simulink model "gm_CustArch_v2_vnl"  (R2020a)
settings: Solver=FixedStepDiscrete  StartTime=0.0  StopTime=840000  RelTol=1e-3
libraries: simulink x172, hdlsllib x102
(part 1 of 4)
settings Model: FPTRunName=FPA_Reference  PacingRate=71  Creator=BuccelliLab  LastModifiedBy=diflo
settings SolverCC: AutoInsertRateTranBlk=on  MinimalZcImpactIntegration=on
settings DataIOCC: LimitDataPoints=on  SaveOutput=off  SaveTime=off  ReturnWorkspaceOutputs=off
settings OptimizationCC: BlockReduction=off  ConditionallyExecuteInputs=off  DefaultParameterBehavior=Inlined  LifeSpan=inf
settings DebuggingCC: SignalRangeChecking=warning  ReadBeforeWriteMsg=DisableAll  WriteAfterWriteMsg=DisableAll  WriteAfterReadMsg=DisableAll  AlgebraicLoopMsg=error  InheritedTsInSrcMsg=none  MultiTaskDSMMsg=none  SingleTaskRateTransMsg=error  ParameterDowncastMsg=warning  ParameterOverflowMsg=warning  AllowSymbolicDim=off  StrictBusMsg=ErrorOnBusTreatedAsVector  SFUnexpectedBacktrackingDiag=warning  SFNoUnconditionalDefaultTransitionDiag=warning  SFExecutionAtInitializationDiag=none  ArithmeticOperatorsInVariantConditions=warning
settings HardwareCC: ProdBitPerPointer=32  ProdBitPerSizeT=32  ProdBitPerPtrDiffT=32  ProdLargestAtomicFloat=None  ProdIntDivRoundTo=Undefined  ProdEndianess=Unspecified  ProdWordSize=32  ProdHWDeviceType=ASIC/FPGA->ASIC/FPGA  TargetBitPerPointer=64  TargetBitPerSizeT=64  TargetBitPerPtrDiffT=64  TargetLongLongMode=on  TargetIntDivRoundTo=Zero  TargetEndianess=LittleEndian  TargetWordSize=64  TargetHWDeviceType=Custom Processor->MATLAB Host Computer  ProdEqTarget=off
settings ModelReferenceCC: UpdateModelReferenceTargets=IfOutOfDate
settings SFSimCC: SFSimEcho=off  SimUseLocalCustomCode=off  CustomCodeUndefinedFunction=UseInterfaceOnly
settings RTWCC: RTWUseLocalCustomCode=off
settings CodeAppCC: StateflowObjectComments=on
settings GRTTargetCC: TargetLangStandard=C89/C90 (ANSI)
settings ConfigComp: CovScope=ReferencedModels  CovMetricSettings=dw  CovHtmlReporting=on  CovSaveCumulativeToWorkspaceVar=on  CovSaveSingleToWorkspaceVar=on  CovExternalEMLEnable=off  CovSFcnEnable=off

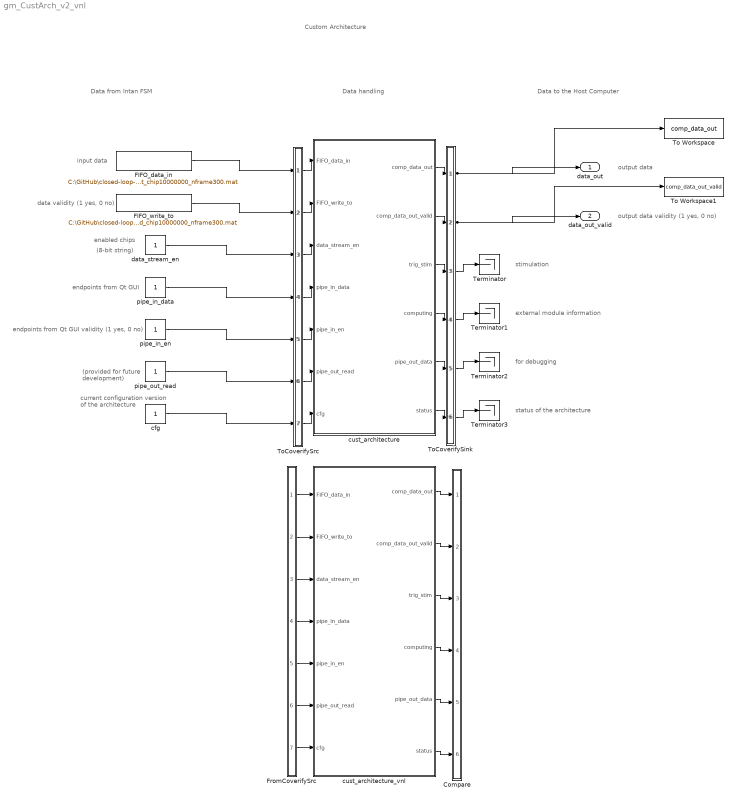
== system gm_CustArch_v2_vnl ==
  note: Data handling
  note: Custom Architecture
  note: output data validity (1 yes, 0 no)
  note: endpoints from Qt GUI
  note: (8-bit string)
  note: enabled chips
  note: data validity (1 yes, 0 no)
  note: input data
  note: endpoints from Qt GUI validity (1 yes, 0 no)
  note: (provided for future
      | development)
  note: current configuration
      | version of the
      | architecture
  note: output data
  note: Data to the Host Computer
  note: stimulation
  note: external module information
  note: for debugging
  note: status of the architecture
  note: Data from Intan FSM
  Compare : Subsystem
      mask Display: disp('')
  FIFO_data_in : FromFile  FileName=C:\GitHub\closed-loop-neuroscience\Mattia\Custom_architecture\CustArch_debug\fsm_out_chip10000000_nframe300.mat  OutDataTypeStr=uint16  SampleTime=1  ExtrapolationBeforeFirstDataPoint=Hold first value  InterpolationWithinTimeRange=Zero order hold  ExtrapolationAfterLastDataPoint=Hold last value
  FIFO_write_to : FromFile  FileName=C:\GitHub\closed-loop-neuroscience\Mattia\Custom_architecture\CustArch_debug\fsm_valid_chip10000000_nframe300.mat  OutDataTypeStr=boolean  SampleTime=1
  FromCoverifySrc : Subsystem
      mask Display: disp('')
  Terminator{,1..3} (4 alike) : Terminator
  To Workspace : ToWorkspace  VariableName=comp_data_out  SaveFormat=Timeseries  SampleTime=-1
  To Workspace1 : ToWorkspace  VariableName=comp_data_out_valid  SaveFormat=Timeseries  SampleTime=-1
  ToCoverifySink : Subsystem
      mask Display: disp('')
  ToCoverifySrc : Subsystem
      mask Display: disp('')
  cfg : Constant  OutDataTypeStr=uint16  SampleTime=-1
  cust_architecture : Subsystem
  cust_architecture_vnl : Subsystem
  data_stream_en : Constant  OutDataTypeStr=uint8  SampleTime=-1
  pipe_in_data : Constant  OutDataTypeStr=uint16  SampleTime=-1
  pipe_in_en : Constant  OutDataTypeStr=boolean  SampleTime=-1
  pipe_out_read : Constant  OutDataTypeStr=boolean  SampleTime=-1
  data_out : Outport  VectorParamsAs1DForOutWhenUnconnected=off
  data_out_valid : Outport  Port=2  VectorParamsAs1DForOutWhenUnconnected=off
  wires:
  ToCoverifySrc/1(out1) -> cust_architecture/1(FIFO_data_in)
  ToCoverifySrc/2(out2) -> cust_architecture/2(FIFO_write_to)
  ToCoverifySrc/3(out3) -> cust_architecture/3(data_stream_en)
  ToCoverifySrc/4(out4) -> cust_architecture/4(pipe_in_data)
  ToCoverifySrc/5(out5) -> cust_architecture/5(pipe_in_en)
  ToCoverifySrc/6(out6) -> cust_architecture/6(pipe_out_read)
  ToCoverifySrc/7(out7) -> cust_architecture/7(cfg)
  cust_architecture/1(comp_data_out) -> ToCoverifySink/1(in1)
  cust_architecture/2(comp_data_out_valid) -> ToCoverifySink/2(in2)
  cust_architecture/3(trig_stim) -> ToCoverifySink/3(in3)
  cust_architecture/4(computing) -> ToCoverifySink/4(in4)
  cust_architecture/5(pipe_out_data) -> ToCoverifySink/5(in5)
  cust_architecture/6(status) -> ToCoverifySink/6(in6)
  FIFO_data_in/1 -> ToCoverifySrc/1(in1)
  FIFO_write_to/1 -> ToCoverifySrc/2(in2)
  data_stream_en/1 -> ToCoverifySrc/3(in3)
  pipe_in_data/1 -> ToCoverifySrc/4(in4)
  pipe_in_en/1 -> ToCoverifySrc/5(in5)
  pipe_out_read/1 -> ToCoverifySrc/6(in6)
  cfg/1 -> ToCoverifySrc/7(in7)
  ToCoverifySink/1(out1) -> data_out/1, To Workspace/1
  ToCoverifySink/2(out2) -> data_out_valid/1, To Workspace1/1
  ToCoverifySink/3(out3) -> Terminator/1
  ToCoverifySink/4(out4) -> Terminator1/1
  ToCoverifySink/5(out5) -> Terminator2/1
  ToCoverifySink/6(out6) -> Terminator3/1
  FromCoverifySrc/1(out1) -> cust_architecture_vnl/1(FIFO_data_in)
  FromCoverifySrc/2(out2) -> cust_architecture_vnl/2(FIFO_write_to)
  FromCoverifySrc/3(out3) -> cust_architecture_vnl/3(data_stream_en)
  FromCoverifySrc/4(out4) -> cust_architecture_vnl/4(pipe_in_data)
  FromCoverifySrc/5(out5) -> cust_architecture_vnl/5(pipe_in_en)
  FromCoverifySrc/6(out6) -> cust_architecture_vnl/6(pipe_out_read)
  FromCoverifySrc/7(out7) -> cust_architecture_vnl/7(cfg)
  cust_architecture_vnl/1(comp_data_out) -> Compare/1(in1)
  cust_architecture_vnl/2(comp_data_out_valid) -> Compare/2(in2)
  cust_architecture_vnl/3(trig_stim) -> Compare/3(in3)
  cust_architecture_vnl/4(computing) -> Compare/4(in4)
  cust_architecture_vnl/5(pipe_out_data) -> Compare/5(in5)
  cust_architecture_vnl/6(status) -> Compare/6(in6)

== system gm_CustArch_v2_vnl/Compare ==
  in1 : Inport
  in2 : Inport  Port=2
  in3 : Inport  Port=3
  in4 : Inport  Port=4
  in5 : Inport  Port=5
  in6 : Inport  Port=6
  Assert_comp_data_out : Subsystem
  Assert_comp_data_out_valid : Subsystem
  Assert_computing : Subsystem
  Assert_pipe_out_data : Subsystem
  Assert_status : Subsystem
  Assert_trig_stim : Subsystem
  CleanupScopes : Subsystem
      settings: OpenFcn=|
      | blkName = gcb; %self block
      | idx = regexp(blkName, '/CleanupScopes$', 'once');
      | blkParent = blkName(1:idx-1);
      | blks=find_system(blkParent, 'LookUnderMasks', 'all','blocktype', 'Scope');
      | for itr = 1:length(blks)
      | 	 hScopeCfg = get_param(blks{itr},'ScopeConfiguration');
      | 	 hScopeCfg.Visible = ~ hScopeCfg.Visible;
      | end
      | drawnow;
      mask Display: fprintf(message('hdlcoder:cosim:vnl_dblclick').getString());
  Enable : Subsystem
      settings: OpenFcn=|
      | blkName = gcb;
      | idx = regexp(blkName, '/Enable$', 'once');
      | blkParent = blkName(1:idx-1);
      | blks=find_system(blkParent, 'LookUnderMasks', 'all','blocktype', 'Assertion');
      | e = get_param(blks{1}, 'Enabled');
      | if strcmp(e, 'on'), f= 'off';, else, f = 'on';, end
      | for ii=1:length(blks), set_param(blks{ii}, 'Enabled', f);, end
      | set_param(gcb, 'MaskDisplay',['fprintf(message(''hdlcoder:cosim:vnl_dblclick_assertions'',','''',upper(e),'''',').getString())']);
      mask Display: fprintf(message('hdlcoder:cosim:vnl_dblclick_assertions','OFF').getString());
  wires:
  in1/1 -> Assert_comp_data_out/1(cosim)
  [out1] -> Assert_comp_data_out/2(dut)
  in2/1 -> Assert_comp_data_out_valid/1(cosim)
  [out2] -> Assert_comp_data_out_valid/2(dut)
  in3/1 -> Assert_trig_stim/1(cosim)
  [out3] -> Assert_trig_stim/2(dut)
  in4/1 -> Assert_computing/1(cosim)
  [out4] -> Assert_computing/2(dut)
  in5/1 -> Assert_pipe_out_data/1(cosim)
  [out5] -> Assert_pipe_out_data/2(dut)
  in6/1 -> Assert_status/1(cosim)
  [out6] -> Assert_status/2(dut)

== system gm_CustArch_v2_vnl/FromCoverifySrc ==
  out1 : Outport
  out2 : Outport  Port=2
  out3 : Outport  Port=3
  out4 : Outport  Port=4
  out5 : Outport  Port=5
  out6 : Outport  Port=6
  out7 : Outport  Port=7
  wires:
  [in1] -> out1/1
  [in2] -> out2/1
  [in3] -> out3/1
  [in4] -> out4/1
  [in5] -> out5/1
  [in6] -> out6/1
  [in7] -> out7/1

== system gm_CustArch_v2_vnl/ToCoverifySink ==
  in1 : Inport
  in2 : Inport  Port=2
  in3 : Inport  Port=3
  in4 : Inport  Port=4
  in5 : Inport  Port=5
  in6 : Inport  Port=6
  out1 : Outport
  out2 : Outport  Port=2
  out3 : Outport  Port=3
  out4 : Outport  Port=4
  out5 : Outport  Port=5
  out6 : Outport  Port=6
  tag scope: out1=global, out2=global, out3=global, out4=global, out5=global, out6=global
  wires:
  in1/1 -> out1/1, [out1]
  in2/1 -> out2/1, [out2]
  in3/1 -> out3/1, [out3]
  in4/1 -> out4/1, [out4]
  in5/1 -> out5/1, [out5]
  in6/1 -> out6/1, [out6]

== system gm_CustArch_v2_vnl/ToCoverifySrc ==
  in1 : Inport
  in2 : Inport  Port=2
  in3 : Inport  Port=3
  in4 : Inport  Port=4
  in5 : Inport  Port=5
  in6 : Inport  Port=6
  in7 : Inport  Port=7
  out1 : Outport
  out2 : Outport  Port=2
  out3 : Outport  Port=3
  out4 : Outport  Port=4
  out5 : Outport  Port=5
  out6 : Outport  Port=6
  out7 : Outport  Port=7
  tag scope: in1=global, in2=global, in3=global, in4=global, in5=global, in6=global, in7=global
  wires:
  in1/1 -> out1/1, [in1]
  in2/1 -> out2/1, [in2]
  in3/1 -> out3/1, [in3]
  in4/1 -> out4/1, [in4]
  in5/1 -> out5/1, [in5]
  in6/1 -> out6/1, [in6]
  in7/1 -> out7/1, [in7]

== system gm_CustArch_v2_vnl/cust_architecture ==
  FIFO_data_in : Inport  OutDataTypeStr=uint16  PortDimensions=1  SampleTime=1
  FIFO_write_to : Inport  Port=2  OutDataTypeStr=boolean  PortDimensions=1  SampleTime=1
  data_stream_en : Inport  Port=3  OutDataTypeStr=uint8  PortDimensions=1  SampleTime=1
  pipe_in_data : Inport  Port=4  OutDataTypeStr=uint16  PortDimensions=1  SampleTime=1
  pipe_in_en : Inport  Port=5  OutDataTypeStr=boolean  PortDimensions=1  SampleTime=1
  pipe_out_read : Inport  Port=6  OutDataTypeStr=boolean  PortDimensions=1  SampleTime=1
  cfg : Inport  Port=7  OutDataTypeStr=uint16  PortDimensions=1  SampleTime=1
  Constant : Constant  OutDataTypeStr=uint8  SampleTime=1
  Constant1 : Constant  OutDataTypeStr=boolean  SampleTime=1
  Constant2 : Constant  OutDataTypeStr=uint16  SampleTime=1
  Constant3 : Constant  OutDataTypeStr=uint16  SampleTime=1
  Terminator2 : Terminator
  Terminator3 : Terminator
  Terminator4 : Terminator
  collect_output : Subsystem
  input_interpret_store_retrieve : Subsystem
  output_interpret : Subsystem
  pipe_in_interpret : Subsystem
  process_and_retrieve : Subsystem
  comp_data_out : Outport  VectorParamsAs1DForOutWhenUnconnected=off
  comp_data_out_valid : Outport  Port=2  OutDataTypeStr=boolean  VectorParamsAs1DForOutWhenUnconnected=off
  trig_stim : Outport  Port=3  VectorParamsAs1DForOutWhenUnconnected=off
  computing : Outport  Port=4  VectorParamsAs1DForOutWhenUnconnected=off
  pipe_out_data : Outport  Port=5  VectorParamsAs1DForOutWhenUnconnected=off
  status : Outport  Port=6  VectorParamsAs1DForOutWhenUnconnected=off
  wires:
  process_and_retrieve/1(rd_dout) -> collect_output/8(rd_dout)
  pipe_in_interpret/1(Out1) -> process_and_retrieve/5(value_from_pipeIn)
  output_interpret/3(read_address) -> input_interpret_store_retrieve/3(read_address), collect_output/6(rd_address)
  output_interpret/2(rd_enable) -> collect_output/5(rd_enable)
  output_interpret/1(OutputState) -> collect_output/4(OutputState)
  input_interpret_store_retrieve/4(read_from_processing_addr) -> process_and_retrieve/4(read_from_processing_addr)
  input_interpret_store_retrieve/3(current_value) -> process_and_retrieve/3(current_value)
  input_interpret_store_retrieve/2(read_from_storage_value) -> collect_output/7(read_from_storage_value)
  input_interpret_store_retrieve/1(InputState) -> process_and_retrieve/2(InputState), output_interpret/2(InputState), collect_output/3(InputState)
  collect_output/3(rd_address_bit_set_AC_during_DC) -> process_and_retrieve/1(rd_address_bit_set_AC_during_DC)
  collect_output/2(comp_data_out) -> comp_data_out/1
  collect_output/1(comp_data_out_valid) -> comp_data_out_valid/1
  Constant3/1 -> status/1
  Constant2/1 -> pipe_out_data/1
  Constant1/1 -> computing/1
  Constant/1 -> trig_stim/1
  cfg/1 -> Terminator2/1
  pipe_out_read/1 -> Terminator3/1
  pipe_in_en/1 -> Terminator4/1
  pipe_in_data/1 -> pipe_in_interpret/1(In1)
  data_stream_en/1 -> input_interpret_store_retrieve/4(data_stream_enable), output_interpret/1(data_stream_enable)
  FIFO_write_to/1 -> input_interpret_store_retrieve/2(FIFO_write_to), collect_output/2(FIFO_write_to)
  FIFO_data_in/1 -> collect_output/1(FIFO_data_in), input_interpret_store_retrieve/1(FIFO_data_in)

== system gm_CustArch_v2_vnl/cust_architecture_vnl ==
  note: Input
  note: Output
  note: Processing
  note: Unused
  FIFO_data_in : Inport
  FIFO_write_to : Inport  Port=2
  data_stream_en : Inport  Port=3
  pipe_in_data : Inport  Port=4
  pipe_in_en : Inport  Port=5
  pipe_out_read : Inport  Port=6
  cfg : Inport  Port=7
  Constant : Constant  OutDataTypeStr=uint8  SampleTime=-1
  Constant1 : Constant  OutDataTypeStr=boolean  SampleTime=-1
  Constant2 : Constant  OutDataTypeStr=uint16  SampleTime=-1
  Constant3 : Constant  OutDataTypeStr=uint16  SampleTime=-1
  Terminator2 : Terminator
  Terminator3 : Terminator
  Terminator4 : Terminator
  collect_output : Subsystem
  input_interpret_store_retrieve : Subsystem
  output_interpret : Subsystem
  pipe_in_interpret : Subsystem
  process_and_retrieve : Subsystem
  comp_data_out : Outport  VectorParamsAs1DForOutWhenUnconnected=off
  comp_data_out_valid : Outport  Port=2  OutDataTypeStr=boolean  VectorParamsAs1DForOutWhenUnconnected=off
  trig_stim : Outport  Port=3  VectorParamsAs1DForOutWhenUnconnected=off
  computing : Outport  Port=4  VectorParamsAs1DForOutWhenUnconnected=off
  pipe_out_data : Outport  Port=5  VectorParamsAs1DForOutWhenUnconnected=off
  status : Outport  Port=6  VectorParamsAs1DForOutWhenUnconnected=off
  wires:
  process_and_retrieve/1(rd_dout) -> collect_output/8(rd_dout)
  pipe_in_interpret/1(Out1) -> process_and_retrieve/5(value_from_pipeIn)
  input_interpret_store_retrieve/4(read_from_processing_addr) -> process_and_retrieve/4(read_from_processing_addr)
  input_interpret_store_retrieve/3(current_value) -> process_and_retrieve/3(current_value)
  collect_output/3(rd_address_bit_set_AC_during_DC) -> process_and_retrieve/1(rd_address_bit_set_AC_during_DC)
  pipe_in_data/1 -> pipe_in_interpret/1(In1)
  output_interpret/2(rd_enable) -> collect_output/5(rd_enable)
  output_interpret/1(OutputState) -> collect_output/4(OutputState)
  output_interpret/3(read_address) -> input_interpret_store_retrieve/3(read_address), collect_output/6(rd_address)
  input_interpret_store_retrieve/2(read_from_storage_value) -> collect_output/7(read_from_storage_value)
  input_interpret_store_retrieve/1(InputState) -> process_and_retrieve/2(InputState), output_interpret/2(InputState), collect_output/3(InputState)
  collect_output/2(comp_data_out) -> comp_data_out/1
  collect_output/1(comp_data_out_valid) -> comp_data_out_valid/1
  pipe_in_en/1 -> Terminator4/1
  pipe_out_read/1 -> Terminator3/1
  cfg/1 -> Terminator2/1
  Constant3/1 -> status/1
  Constant2/1 -> pipe_out_data/1
  Constant1/1 -> computing/1
  Constant/1 -> trig_stim/1
  data_stream_en/1 -> input_interpret_store_retrieve/4(data_stream_enable), output_interpret/1(data_stream_enable)
  FIFO_write_to/1 -> input_interpret_store_retrieve/2(FIFO_write_to), collect_output/2(FIFO_write_to)
  FIFO_data_in/1 -> collect_output/1(FIFO_data_in), input_interpret_store_retrieve/1(FIFO_data_in)

== system gm_CustArch_v2_vnl/Compare/Assert_comp_data_out ==
  cosim : Inport
  dut : Inport  Port=2
  AssertEq : Assertion  StopWhenAssertionFail=off
  Compare To Zero : simulink/Logic and Bit Operations/Compare To Zero  relop===  OutDataTypeStr=boolean
  Relational Operator : RelationalOperator  Operator===  OutDataTypeStr=boolean  RndMeth=Nearest
  compare: comp_data_out : Scope  NumInputPorts=3
  wires:
  Compare To Zero/1 -> compare: comp_data_out/3  "err"
  Relational Operator/1 -> Compare To Zero/1, AssertEq/1
  cosim/1 -> compare: comp_data_out/1, Relational Operator/1  "cosim"
  dut/1 -> compare: comp_data_out/2, Relational Operator/2  "dut ref"

== system gm_CustArch_v2_vnl/Compare/Assert_comp_data_out_valid ==
  cosim : Inport
  dut : Inport  Port=2
  AssertEq : Assertion  StopWhenAssertionFail=off
  Compare To Zero : simulink/Logic and Bit Operations/Compare To Zero  relop===  OutDataTypeStr=boolean
  Relational Operator : RelationalOperator  Operator===  OutDataTypeStr=boolean  RndMeth=Nearest
  compare: comp_data_out_valid : Scope  NumInputPorts=3
  wires:
  Compare To Zero/1 -> compare: comp_data_out_valid/3  "err"
  Relational Operator/1 -> Compare To Zero/1, AssertEq/1
  cosim/1 -> compare: comp_data_out_valid/1, Relational Operator/1  "cosim"
  dut/1 -> compare: comp_data_out_valid/2, Relational Operator/2  "dut ref"

== system gm_CustArch_v2_vnl/Compare/Assert_computing ==
  cosim : Inport
  dut : Inport  Port=2
  AssertEq : Assertion  StopWhenAssertionFail=off
  Compare To Zero : simulink/Logic and Bit Operations/Compare To Zero  relop===  OutDataTypeStr=boolean
  Relational Operator : RelationalOperator  Operator===  OutDataTypeStr=boolean  RndMeth=Nearest
  compare: computing : Scope  NumInputPorts=3
  wires:
  Compare To Zero/1 -> compare: computing/3  "err"
  Relational Operator/1 -> Compare To Zero/1, AssertEq/1
  cosim/1 -> compare: computing/1, Relational Operator/1  "cosim"
  dut/1 -> compare: computing/2, Relational Operator/2  "dut ref"

== system gm_CustArch_v2_vnl/Compare/Assert_pipe_out_data ==
  cosim : Inport
  dut : Inport  Port=2
  AssertEq : Assertion  StopWhenAssertionFail=off
  Compare To Zero : simulink/Logic and Bit Operations/Compare To Zero  relop===  OutDataTypeStr=boolean
  Relational Operator : RelationalOperator  Operator===  OutDataTypeStr=boolean  RndMeth=Nearest
  compare: pipe_out_data : Scope  NumInputPorts=3
  wires:
  Compare To Zero/1 -> compare: pipe_out_data/3  "err"
  Relational Operator/1 -> Compare To Zero/1, AssertEq/1
  cosim/1 -> compare: pipe_out_data/1, Relational Operator/1  "cosim"
  dut/1 -> compare: pipe_out_data/2, Relational Operator/2  "dut ref"

== system gm_CustArch_v2_vnl/Compare/Assert_status ==
  cosim : Inport
  dut : Inport  Port=2
  AssertEq : Assertion  StopWhenAssertionFail=off
  Compare To Zero : simulink/Logic and Bit Operations/Compare To Zero  relop===  OutDataTypeStr=boolean
  Relational Operator : RelationalOperator  Operator===  OutDataTypeStr=boolean  RndMeth=Nearest
  compare: status : Scope  NumInputPorts=3
  wires:
  Compare To Zero/1 -> compare: status/3  "err"
  Relational Operator/1 -> Compare To Zero/1, AssertEq/1
  cosim/1 -> compare: status/1, Relational Operator/1  "cosim"
  dut/1 -> compare: status/2, Relational Operator/2  "dut ref"

== system gm_CustArch_v2_vnl/Compare/Assert_trig_stim ==
  cosim : Inport
  dut : Inport  Port=2
  AssertEq : Assertion  StopWhenAssertionFail=off
  Compare To Zero : simulink/Logic and Bit Operations/Compare To Zero  relop===  OutDataTypeStr=boolean
  Relational Operator : RelationalOperator  Operator===  OutDataTypeStr=boolean  RndMeth=Nearest
  compare: trig_stim : Scope  NumInputPorts=3
  wires:
  Compare To Zero/1 -> compare: trig_stim/3  "err"
  Relational Operator/1 -> Compare To Zero/1, AssertEq/1
  cosim/1 -> compare: trig_stim/1, Relational Operator/1  "cosim"
  dut/1 -> compare: trig_stim/2, Relational Operator/2  "dut ref"

== system gm_CustArch_v2_vnl/Compare/CleanupScopes ==

== system gm_CustArch_v2_vnl/Compare/Enable ==

== system gm_CustArch_v2_vnl/cust_architecture/collect_output ==
  FIFO_data_in : Inport  OutDataTypeStr=uint16  PortDimensions=1  SampleTime=1
  FIFO_write_to : Inport  Port=2  OutDataTypeStr=boolean  PortDimensions=1  SampleTime=1
  InputState : Inport  Port=3  OutDataTypeStr=uint8  PortDimensions=1  SampleTime=1
  OutputState : Inport  Port=4  OutDataTypeStr=uint8  PortDimensions=1  SampleTime=1
  rd_enable : Inport  Port=5  OutDataTypeStr=boolean  PortDimensions=1  SampleTime=1
  rd_address : Inport  Port=6  OutDataTypeStr=fixdt(0, 9, 0)  PortDimensions=1  SampleTime=1
  read_from_storage_value : Inport  Port=7  OutDataTypeStr=uint16  PortDimensions=1  SampleTime=1
  rd_dout : Inport  Port=8  OutDataTypeStr=uint16  PortDimensions=1  SampleTime=1
  AND : Logic  AllPortsSameDT=off  OutDataTypeStr=boolean  SampleTime=1
  Bit Set to get AC during DC : simulink/Logic and Bit Operations/Bit Set  iBit=0
      settings: SourceProductBaseCode=SL
  Compare To Constant : simulink/Logic and Bit Operations/Compare To Constant  relop=<  const="fi(0,0,8,0,\"hex\",\"06\")"  OutDataTypeStr=boolean
  Memory : UnitDelay  InitialCondition=double(0)  SampleTime=1
  Memory1 : UnitDelay  InitialCondition=double(0)  SampleTime=1
  Memory7 : UnitDelay  InitialCondition=double(0)  SampleTime=1
  Switch : Switch  Criteria=u2 > Threshold  Threshold=double(0)  OutDataTypeStr=uint16  SampleTime=1
  Switch2 : Switch  Criteria=u2 > Threshold  Threshold=double(0)  OutDataTypeStr=uint16  SampleTime=1
  get_data_only_when_enabled : Subsystem
  output_state_DC : simulink/Logic and Bit Operations/Compare To Constant  relop=~=  const="fi(0,0,8,0,\"hex\",\"06\")"  OutDataTypeStr=boolean
  read_from_magic_and_timestamp : Subsystem
  comp_data_out_valid : Outport
  comp_data_out : Outport  Port=2
  rd_address_bit_set_AC_during_DC : Outport  Port=3
  wires:
  read_from_magic_and_timestamp/1(read_from_Magic_TS) -> Switch/1
  output_state_DC/1 -> Memory7/1
  get_data_only_when_enabled/1(Out1) -> comp_data_out/1
  Switch2/1 -> Switch/3
  Switch/1 -> get_data_only_when_enabled/1(In1)
  Memory7/1 -> Switch2/2
  Memory1/1 -> get_data_only_when_enabled/Enable, comp_data_out_valid/1, AND/2
  Memory/1 -> Compare To Constant/1
  Compare To Constant/1 -> AND/1
  Bit Set to get AC during DC/1 -> rd_address_bit_set_AC_during_DC/1
  AND/1 -> Switch/2
  rd_dout/1 -> Switch2/3
  read_from_storage_value/1 -> Switch2/1
  rd_address/1 -> Bit Set to get AC during DC/1
  rd_enable/1 -> Memory1/1
  OutputState/1 -> read_from_magic_and_timestamp/1(OutputState), Memory/1, output_state_DC/1
  InputState/1 -> read_from_magic_and_timestamp/4(InputState)
  FIFO_write_to/1 -> read_from_magic_and_timestamp/3(FIFO_write_to)
  FIFO_data_in/1 -> read_from_magic_and_timestamp/2(FIFO_data_in)

== system gm_CustArch_v2_vnl/cust_architecture/input_interpret_store_retrieve ==
  note: data sent to Output
  note: data sent for processing
  note: address sent for processing
  FIFO_data_in : Inport  OutDataTypeStr=uint16  PortDimensions=1  SampleTime=1
  FIFO_write_to : Inport  Port=2  OutDataTypeStr=boolean  PortDimensions=1  SampleTime=1
  read_address : Inport  Port=3  OutDataTypeStr=fixdt(0, 9, 0)  PortDimensions=1  SampleTime=1
  data_stream_enable : Inport  Port=4  OutDataTypeStr=uint8  PortDimensions=1  SampleTime=1
  InputStateMachine : Subsystem
  Interpret_to_RAM_input : Subsystem
  store_and_retrieve_input : Subsystem
  InputState : Outport
  read_from_storage_value : Outport  Port=2
  current_value : Outport  Port=3
  read_from_processing_addr : Outport  Port=4
  wires:
  store_and_retrieve_input/3(read_from_porcessing_addr) -> read_from_processing_addr/1
  store_and_retrieve_input/2(current_value) -> current_value/1
  store_and_retrieve_input/1(read_from_storage_value) -> read_from_storage_value/1
  Interpret_to_RAM_input/5(wr_en) -> store_and_retrieve_input/4(wr_en)
  Interpret_to_RAM_input/4(write address) -> store_and_retrieve_input/3(wr_address)
  Interpret_to_RAM_input/3(wr_din) -> store_and_retrieve_input/2(wr_din)
  Interpret_to_RAM_input/2(inc_source_device) -> InputStateMachine/4(inc_source_device_MSB)
  Interpret_to_RAM_input/1(device_output) -> InputStateMachine/3(channel_0_19)
  InputStateMachine/1(InputState) -> Interpret_to_RAM_input/3(InputState), InputState/1
  data_stream_enable/1 -> Interpret_to_RAM_input/4(data_stream_enable)
  read_address/1 -> store_and_retrieve_input/1(read address)
  FIFO_write_to/1 -> Interpret_to_RAM_input/2(FIFO_write_to), InputStateMachine/2(FIFO_write_to)
  FIFO_data_in/1 -> Interpret_to_RAM_input/1(FIFO_data_in), InputStateMachine/1(FIFO_data_in)

== system gm_CustArch_v2_vnl/cust_architecture/output_interpret ==
  data_stream_enable : Inport  OutDataTypeStr=uint8  PortDimensions=1  SampleTime=1
  InputState : Inport  Port=2  OutDataTypeStr=uint8  PortDimensions=1  SampleTime=1
  Interpret_to_RAM_output : Subsystem
  OutputStateMachine : Subsystem
  OutputState : Outport
  rd_enable : Outport  Port=2
  read_address : Outport  Port=3
  wires:
  OutputStateMachine/1(OutputState) -> Interpret_to_RAM_output/1(OutputState), OutputState/1
  Interpret_to_RAM_output/2(read address) -> read_address/1
  Interpret_to_RAM_output/1(rd_enable) -> rd_enable/1
  InputState/1 -> OutputStateMachine/1(input_state)
  data_stream_enable/1 -> Interpret_to_RAM_output/2(data_stream_en)

== system gm_CustArch_v2_vnl/cust_architecture/pipe_in_interpret ==
  In1 : Inport  OutDataTypeStr=uint16  PortDimensions=1  SampleTime=1
  Bit Slice1 : hdlsllib/Logic and Bit Operations/Bit Slice  lidx=double(15)  ridx=double(8)
      settings: SourceProductBaseCode=SL
  Compare To Constant1 : simulink/Logic and Bit Operations/Compare To Constant  relop===  const="fi(0,0,8,0,\"hex\",\"02\")"  OutDataTypeStr=boolean
  Constant4 : Constant  Value=5  OutDataTypeStr=uint16  SampleTime=1
  Memory6 : UnitDelay  InitialCondition=double(0)  SampleTime=1
  Switch1 : Switch  Criteria=u2 > Threshold  Threshold=double(0)  OutDataTypeStr=uint16  SampleTime=1
  Out1 : Outport
  wires:
  Switch1/1 -> Out1/1
  Memory6/1 -> Bit Slice1/1
  Constant4/1 -> Switch1/3
  Compare To Constant1/1 -> Switch1/2
  Bit Slice1/1 -> Compare To Constant1/1
  In1/1 -> Memory6/1, Switch1/1

== system gm_CustArch_v2_vnl/cust_architecture/process_and_retrieve ==
  note: address sent for processing
  note: data sent for processing
  note: rd_address from Output
  note: data processed for Output
  rd_address_bit_set_AC_during_DC : Inport  OutDataTypeStr=fixdt(0, 9, 0)  PortDimensions=1  SampleTime=1
  InputState : Inport  Port=2  OutDataTypeStr=uint8  PortDimensions=1  SampleTime=1
  current_value : Inport  Port=3  OutDataTypeStr=uint16  PortDimensions=1  SampleTime=1
  read_from_processing_addr : Inport  Port=4  OutDataTypeStr=fixdt(0, 9, 0)  PortDimensions=1  SampleTime=1
  value_from_pipeIn : Inport  Port=5  OutDataTypeStr=uint16  PortDimensions=1  SampleTime=1
  DCtoAC_storage : hdlsllib/HDL RAMs/Dual Port RAM  ram_size=9
      settings: SourceProductBaseCode=SL
  Memory2 : UnitDelay  InitialCondition=double(0)  SampleTime=1
  Memory3 : UnitDelay  InitialCondition=double(0)  SampleTime=1
  Memory5 : UnitDelay  InitialCondition=double(0)  SampleTime=1
  Terminator : Terminator
  Terminator7 : Terminator
  input_state_AC : simulink/Logic and Bit Operations/Compare To Constant  relop===  const="fi(0,0,8,0,\"hex\",\"07\")"  OutDataTypeStr=boolean
  rd_dout : Outport
  wires:
  input_state_AC/1 -> Memory2/1
  Memory5/1 -> DCtoAC_storage/2
  Memory3/1 -> input_state_AC/1
  Memory2/1 -> DCtoAC_storage/3
  DCtoAC_storage/2 -> rd_dout/1
  DCtoAC_storage/1 -> Terminator7/1
  value_from_pipeIn/1 -> Terminator/1
  read_from_processing_addr/1 -> Memory5/1
  current_value/1 -> DCtoAC_storage/1
  InputState/1 -> Memory3/1
  rd_address_bit_set_AC_during_DC/1 -> DCtoAC_storage/4

== system gm_CustArch_v2_vnl/cust_architecture_vnl/collect_output ==
  note: Get data from this or that ram depending on output_state
  note: memorie per temporizzazione per ritardo delle ramp input
      | vale per tutte
  note: if OutputState < 6 e read_enable = 1 --> output magic/timestamp
      | else if OutputState ~= 6 read from storage
      | else read processed data
  note: during the processing step the processed data
      | are saved in the RAM address of the DC data,
      | thus offline it will be possible to compare AC raw
      | and AC filtered data
  FIFO_data_in : Inport
  FIFO_write_to : Inport  Port=2
  InputState : Inport  Port=3
  OutputState : Inport  Port=4
  rd_enable : Inport  Port=5
  rd_address : Inport  Port=6
  read_from_storage_value : Inport  Port=7
  rd_dout : Inport  Port=8
  AND : Logic  IconShape=distinctive  AllPortsSameDT=off  OutDataTypeStr=boolean
  Bit Set to get AC during DC : simulink/Logic and Bit Operations/Bit Set  iBit=0
      settings: SourceProductBaseCode=SL
  Compare To Constant : simulink/Logic and Bit Operations/Compare To Constant  relop=<  const=6  OutDataTypeStr=boolean
  Memory : Memory  InheritSampleTime=on
  Memory1 : Memory  InheritSampleTime=on
  Memory7 : Memory  InheritSampleTime=on
  Switch : Switch  Criteria=u2 > Threshold
  Switch2 : Switch  Criteria=u2 > Threshold
  get_data_only_when_enabled : Subsystem  TreatAsAtomicUnit=on
  output_state_DC : simulink/Logic and Bit Operations/Compare To Constant  relop=~=  const=6  OutDataTypeStr=boolean
  read_from_magic_and_timestamp : Subsystem
  comp_data_out_valid : Outport
  comp_data_out : Outport  Port=2
  rd_address_bit_set_AC_during_DC : Outport  Port=3
  wires:
  InputState/1 -> read_from_magic_and_timestamp/4(InputState)
  FIFO_write_to/1 -> read_from_magic_and_timestamp/3(FIFO_write_to)
  rd_enable/1 -> Memory1/1
  rd_dout/1 -> Switch2/3
  Bit Set to get AC during DC/1 -> rd_address_bit_set_AC_during_DC/1
  OutputState/1 -> Memory/1, read_from_magic_and_timestamp/1(OutputState), output_state_DC/1
  read_from_magic_and_timestamp/1(read_from_Magic_TS) -> Switch/1
  Memory7/1 -> Switch2/2
  Compare To Constant/1 -> AND/1
  output_state_DC/1 -> Memory7/1
  Switch2/1 -> Switch/3  "read_from_storage"
  AND/1 -> Switch/2
  Switch/1 -> get_data_only_when_enabled/1(In1)
  Memory1/1 -> get_data_only_when_enabled/Enable, comp_data_out_valid/1, AND/2
  Memory/1 -> Compare To Constant/1
  rd_address/1 -> Bit Set to get AC during DC/1
  read_from_storage_value/1 -> Switch2/1
  FIFO_data_in/1 -> read_from_magic_and_timestamp/2(FIFO_data_in)
  get_data_only_when_enabled/1(Out1) -> comp_data_out/1  "read_from_storage_post"

== system gm_CustArch_v2_vnl/cust_architecture_vnl/input_interpret_store_retrieve ==
  note: reading address
      | from output
  note: address sent for processing
  note: data sent for processing
  note: data sent to Output
  FIFO_data_in : Inport
  FIFO_write_to : Inport  Port=2
  read_address : Inport  Port=3
  data_stream_enable : Inport  Port=4
  InputStateMachine : Stateflow chart  TreatAsAtomicUnit=on
  Interpret_to_RAM_input : Subsystem
  store_and_retrieve_input : Subsystem
  InputState : Outport
  read_from_storage_value : Outport  Port=2
  current_value : Outport  Port=3
  read_from_processing_addr : Outport  Port=4
  wires:
  store_and_retrieve_input/2(current_value) -> current_value/1
  store_and_retrieve_input/3(read_from_porcessing_addr) -> read_from_processing_addr/1
  data_stream_enable/1 -> Interpret_to_RAM_input/4(data_stream_enable)
  read_address/1 -> store_and_retrieve_input/1(read address)
  FIFO_write_to/1 -> InputStateMachine/2(FIFO_write_to), Interpret_to_RAM_input/2(FIFO_write_to)
  FIFO_data_in/1 -> Interpret_to_RAM_input/1(FIFO_data_in), InputStateMachine/1(FIFO_data_in)
  Interpret_to_RAM_input/3(wr_din) -> store_and_retrieve_input/2(wr_din)
  Interpret_to_RAM_input/1(device_output) -> InputStateMachine/3(channel_0_19)
  Interpret_to_RAM_input/2(inc_source_device) -> InputStateMachine/4(inc_source_device_MSB)
  store_and_retrieve_input/1(read_from_storage_value) -> read_from_storage_value/1
  InputStateMachine/1(InputState) -> Interpret_to_RAM_input/3(InputState), InputState/1  "InputState"
  Interpret_to_RAM_input/5(wr_en) -> store_and_retrieve_input/4(wr_en)
  Interpret_to_RAM_input/4(write address) -> store_and_retrieve_input/3(wr_address)

== system gm_CustArch_v2_vnl/cust_architecture_vnl/output_interpret ==
  note: if InputState == 8 I have processed all the 20 channels (16ch + 4aux)
      | and I start with the output encoding
  data_stream_enable : Inport
  InputState : Inport  Port=2
  Interpret_to_RAM_output : Subsystem
  OutputStateMachine : Stateflow chart  TreatAsAtomicUnit=on
  OutputState : Outport
  rd_enable : Outport  Port=2
  read_address : Outport  Port=3
  wires:
  Interpret_to_RAM_output/2(read address) -> read_address/1
  InputState/1 -> OutputStateMachine/1(input_state)
  data_stream_enable/1 -> Interpret_to_RAM_output/2(data_stream_en)
  Interpret_to_RAM_output/1(rd_enable) -> rd_enable/1
  OutputStateMachine/1(OutputState) -> Interpret_to_RAM_output/1(OutputState), OutputState/1  "OutputState"

== system gm_CustArch_v2_vnl/cust_architecture_vnl/pipe_in_interpret ==
  In1 : Inport
  Bit Slice1 : hdlsllib/Logic and Bit Operations/Bit Slice  lidx=15  ridx=8
      settings: SourceProductBaseCode=SL
  Compare To Constant1 : simulink/Logic and Bit Operations/Compare To Constant  relop===  const=2  OutDataTypeStr=boolean
  Constant4 : Constant  Value=5  OutDataTypeStr=uint16  SampleTime=-1
  Memory6 : Memory  InheritSampleTime=on
  Switch1 : Switch  Criteria=u2 > Threshold
  Out1 : Outport
  wires:
  In1/1 -> Memory6/1, Switch1/1
  Constant4/1 -> Switch1/3
  Switch1/1 -> Out1/1
  Compare To Constant1/1 -> Switch1/2
  Memory6/1 -> Bit Slice1/1
  Bit Slice1/1 -> Compare To Constant1/1

== system gm_CustArch_v2_vnl/cust_architecture_vnl/process_and_retrieve ==
  note: address sent for processing
  note: data sent for processing
  note: Note: If a read operation occurs simultaneously at the same address
      | as a write operation, old data appears at the read output port (rd_dout).
  note: note that these RAM are too big.. I just need 160 and thus a reduced address port width
  note: this memory is to guarantee that the input is already stored
  note: Write in RAM only if an AC data
      | is available
  note: rd_address from Output
  note: data processed for Output
  note: generally, all sample in the processing subsystem
      | are delayed by two samples --> the memories are
      | needed for this reason
  note: The dual-port RAM in the input interpret subsystem introduces
      | a sample of delay. Furthermore, I need one sample more of delay
      | due to the IIR filter --> overall delay of two samples
  note: memory for saving AC filtered data in the DC
      | address for the next offline comparison
  rd_address_bit_set_AC_during_DC : Inport
  InputState : Inport  Port=2
  current_value : Inport  Port=3
  read_from_processing_addr : Inport  Port=4
  value_from_pipeIn : Inport  Port=5
  DCtoAC_storage : hdlsllib/HDL RAMs/Dual Port RAM  ram_size=9
      settings: SourceProductBaseCode=SL
  Memory2 : Memory  InheritSampleTime=on
  Memory3 : Memory  InheritSampleTime=on
  Memory5 : Memory  InheritSampleTime=on
  Terminator : Terminator
  Terminator7 : Terminator
  input_state_AC : simulink/Logic and Bit Operations/Compare To Constant  relop===  const=7  OutDataTypeStr=boolean
  rd_dout : Outport
  wires:
  current_value/1 -> DCtoAC_storage/1
  DCtoAC_storage/2 -> rd_dout/1
  read_from_processing_addr/1 -> Memory5/1  "read_from_processing_addr"
  value_from_pipeIn/1 -> Terminator/1
  InputState/1 -> Memory3/1
  Memory3/1 -> input_state_AC/1
  Memory5/1 -> DCtoAC_storage/2  "write porcessing addr = read from storage addr +1"
  input_state_AC/1 -> Memory2/1  "input_state_AC"
  Memory2/1 -> DCtoAC_storage/3
  rd_address_bit_set_AC_during_DC/1 -> DCtoAC_storage/4  "rd_address_bit_set_AC_during_DC"
  DCtoAC_storage/1 -> Terminator7/1

== system gm_CustArch_v2_vnl/cust_architecture/collect_output/get_data_only_when_enabled ==
  In1 : Inport  OutDataTypeStr=uint16  PortDimensions=1  SampleTime=1
  Enable : EnablePort  OutDataTypeStr=boolean
  Out1 : Outport  InitialOutput=0  VectorParamsAs1DForOutWhenUnconnected=off
  wires:
  In1/1 -> Out1/1

== system gm_CustArch_v2_vnl/cust_architecture/collect_output/read_from_magic_and_timestamp ==
  OutputState : Inport  OutDataTypeStr=uint8  PortDimensions=1  SampleTime=1
  FIFO_data_in : Inport  Port=2  OutDataTypeStr=uint16  PortDimensions=1  SampleTime=1
  FIFO_write_to : Inport  Port=3  OutDataTypeStr=boolean  PortDimensions=1  SampleTime=1
  InputState : Inport  Port=4  OutDataTypeStr=uint8  PortDimensions=1  SampleTime=1
  Terminator1 : Terminator
  getting address and enable for Magic and Timestamps : Subsystem
  input_RAM_for_MagicNumber_TimeStamps : hdlsllib/HDL RAMs/Dual Port RAM  ram_size=8
      settings: SourceProductBaseCode=SL
  read_from_Magic_TS : Outport
  wires:
  input_RAM_for_MagicNumber_TimeStamps/2 -> read_from_Magic_TS/1
  input_RAM_for_MagicNumber_TimeStamps/1 -> Terminator1/1
  getting address and enable for Magic and Timestamps/2(wr_enable) -> input_RAM_for_MagicNumber_TimeStamps/3
  getting address and enable for Magic and Timestamps/1(wr_address) -> input_RAM_for_MagicNumber_TimeStamps/2
  InputState/1 -> getting address and enable for Magic and Timestamps/1(InputState)
  FIFO_write_to/1 -> getting address and enable for Magic and Timestamps/2(FIFO_write_to)
  FIFO_data_in/1 -> input_RAM_for_MagicNumber_TimeStamps/1
  OutputState/1 -> input_RAM_for_MagicNumber_TimeStamps/4

== system gm_CustArch_v2_vnl/cust_architecture/input_interpret_store_retrieve/InputStateMachine ==
  FIFO_data_in : Inport  OutDataTypeStr=uint16  PortDimensions=1  SampleTime=1
  FIFO_write_to : Inport  Port=2  OutDataTypeStr=boolean  PortDimensions=1  SampleTime=1
  channel_0_19 : Inport  Port=3  OutDataTypeStr=uint8  PortDimensions=1  SampleTime=1
  inc_source_device_MSB : Inport  Port=4  OutDataTypeStr=boolean  PortDimensions=1  SampleTime=1
  InputStateMachine : Stateflow chart  TreatAsAtomicUnit=on
  InputState : Outport  VectorParamsAs1DForOutWhenUnconnected=off
  wires:
  InputStateMachine/1(InputState) -> InputState/1
  inc_source_device_MSB/1 -> InputStateMachine/4(inc_source_device_MSB)
  channel_0_19/1 -> InputStateMachine/3(channel_0_19)
  FIFO_write_to/1 -> InputStateMachine/2(FIFO_write_to)
  FIFO_data_in/1 -> InputStateMachine/1(FIFO_data_in)

== system gm_CustArch_v2_vnl/cust_architecture/input_interpret_store_retrieve/Interpret_to_RAM_input ==
  FIFO_data_in : Inport  OutDataTypeStr=uint16  PortDimensions=1  SampleTime=1
  FIFO_write_to : Inport  Port=2  OutDataTypeStr=boolean  PortDimensions=1  SampleTime=1
  InputState : Inport  Port=3  OutDataTypeStr=uint8  PortDimensions=1  SampleTime=1
  data_stream_enable : Inport  Port=4  OutDataTypeStr=uint8  PortDimensions=1  SampleTime=1
  RAM address definition : Subsystem
  interpret incoming data : Subsystem
  device_output : Outport
  inc_source_device : Outport  Port=2
  wr_din : Outport  Port=3
  write address : Outport  Port=4
  wr_en : Outport  Port=5
  wires:
  interpret incoming data/5(converter_cnt) -> RAM address definition/5(converter_cnt)
  interpret incoming data/4(source_channel_0_159) -> RAM address definition/3(source_channel_0_159)
  interpret incoming data/3(device_output) -> device_output/1
  interpret incoming data/2(inc_source_device) -> inc_source_device/1
  interpret incoming data/1(source_device) -> RAM address definition/4(source_device)
  RAM address definition/3(write_enable_6to15) -> wr_en/1
  RAM address definition/2(wr_addr) -> write address/1
  RAM address definition/1(wr_din) -> wr_din/1
  data_stream_enable/1 -> interpret incoming data/3(data_stream_enable)
  InputState/1 -> interpret incoming data/2(InputState), RAM address definition/2(InputState)
  FIFO_write_to/1 -> interpret incoming data/1(FIFO_write_to), RAM address definition/6(write_to)
  FIFO_data_in/1 -> RAM address definition/1(DataIn)

== system gm_CustArch_v2_vnl/cust_architecture/input_interpret_store_retrieve/store_and_retrieve_input ==
  note: data sent to Output
  note: writing address
  note: current data
  note: current data
  note: data sent for processing
  note: address sent for processing
  read address : Inport  OutDataTypeStr=fixdt(0, 9, 0)  PortDimensions=1  SampleTime=1
  wr_din : Inport  Port=2  OutDataTypeStr=uint16  PortDimensions=1  SampleTime=1
  wr_address : Inport  Port=3  OutDataTypeStr=fixdt(0, 9, 0)  PortDimensions=1  SampleTime=1
  wr_en : Inport  Port=4  OutDataTypeStr=boolean  PortDimensions=1  SampleTime=1
  Memory4 : UnitDelay  InitialCondition=double(0)  SampleTime=1
  Terminator : Terminator
  Terminator6 : Terminator
  input_storage : hdlsllib/HDL RAMs/Dual Port RAM  ram_size=9
      settings: SourceProductBaseCode=SL
  input_storage_for_processing : hdlsllib/HDL RAMs/Dual Port RAM  ram_size=9
      settings: SourceProductBaseCode=SL
  read_from_storage_value : Outport
  current_value : Outport  Port=2
  read_from_porcessing_addr : Outport  Port=3
  wires:
  input_storage_for_processing/2 -> current_value/1
  input_storage_for_processing/1 -> Terminator6/1
  input_storage/2 -> read_from_storage_value/1
  input_storage/1 -> Terminator/1
  Memory4/1 -> input_storage_for_processing/4, read_from_porcessing_addr/1
  wr_en/1 -> input_storage_for_processing/3, input_storage/3
  wr_address/1 -> input_storage_for_processing/2, input_storage/2, Memory4/1
  wr_din/1 -> input_storage_for_processing/1, input_storage/1
  read address/1 -> input_storage/4

== system gm_CustArch_v2_vnl/cust_architecture/output_interpret/Interpret_to_RAM_output ==
  OutputState : Inport  OutDataTypeStr=uint8  PortDimensions=1  SampleTime=1
  data_stream_en : Inport  Port=2  OutDataTypeStr=uint8  PortDimensions=1  SampleTime=1
  Output_State_to_RAM_address (to read) : Subsystem
  "get_enabled_timings " : Subsystem
  rd_enable : Outport
  read address : Outport  Port=2
  wires:
  "get_enabled_timings "/5(converter_cnt) -> Output_State_to_RAM_address (to read)/6(converter_cnt)
  "get_enabled_timings "/4(source_device) -> Output_State_to_RAM_address (to read)/5(source_device)
  "get_enabled_timings "/3(source_device_enabled) -> Output_State_to_RAM_address (to read)/4(source_device_en)
  "get_enabled_timings "/2(source_channel_0_159) -> Output_State_to_RAM_address (to read)/2(source_channel_0_159)
  "get_enabled_timings "/1(source_channel_en) -> Output_State_to_RAM_address (to read)/1(source_channel_en)
  Output_State_to_RAM_address (to read)/2(rd_addr) -> read address/1
  Output_State_to_RAM_address (to read)/1(rd_enable) -> rd_enable/1
  data_stream_en/1 -> "get_enabled_timings "/2(data_stream_en)
  OutputState/1 -> "get_enabled_timings "/1(OutputState), Output_State_to_RAM_address (to read)/3(OutputState)

== system gm_CustArch_v2_vnl/cust_architecture/output_interpret/OutputStateMachine ==
  input_state : Inport  OutDataTypeStr=uint8  PortDimensions=1  SampleTime=1
  OutputStateMachine : Stateflow chart  TreatAsAtomicUnit=on
  OutputState : Outport  VectorParamsAs1DForOutWhenUnconnected=off
  wires:
  OutputStateMachine/1(OutputState) -> OutputState/1
  input_state/1 -> OutputStateMachine/1(input_state)

== system gm_CustArch_v2_vnl/cust_architecture_vnl/collect_output/get_data_only_when_enabled ==
  In1 : Inport
  Enable : EnablePort
  Out1 : Outport  InitialOutput=0  VectorParamsAs1DForOutWhenUnconnected=off
  wires:
  In1/1 -> Out1/1

== system gm_CustArch_v2_vnl/cust_architecture_vnl/collect_output/read_from_magic_and_timestamp ==
  note: This subsystem in needed for save in a specific RAM the magic number
      | and the timestamp
  OutputState : Inport
  FIFO_data_in : Inport  Port=2
  FIFO_write_to : Inport  Port=3
  InputState : Inport  Port=4
  Terminator1 : Terminator
  getting address and enable for Magic and Timestamps : Subsystem
  input_RAM_for_MagicNumber_TimeStamps : hdlsllib/HDL RAMs/Dual Port RAM  ram_size=8
      settings: SourceProductBaseCode=SL
  read_from_Magic_TS : Outport
  wires:
  FIFO_write_to/1 -> getting address and enable for Magic and Timestamps/2(FIFO_write_to)
  InputState/1 -> getting address and enable for Magic and Timestamps/1(InputState)
  OutputState/1 -> input_RAM_for_MagicNumber_TimeStamps/4
  input_RAM_for_MagicNumber_TimeStamps/1 -> Terminator1/1
  getting address and enable for Magic and Timestamps/1(wr_address) -> input_RAM_for_MagicNumber_TimeStamps/2
  input_RAM_for_MagicNumber_TimeStamps/2 -> read_from_Magic_TS/1  "read_from_Magic_TS"
  getting address and enable for Magic and Timestamps/2(wr_enable) -> input_RAM_for_MagicNumber_TimeStamps/3
  FIFO_data_in/1 -> input_RAM_for_MagicNumber_TimeStamps/1

== system gm_CustArch_v2_vnl/cust_architecture_vnl/input_interpret_store_retrieve/Interpret_to_RAM_input ==
  note: These subsystems identify the sources of the incoming data (amplifier --> source_device and channel number) and
      | determine the address to be associated to the current data for the RAM storage. This statement is valid for all the kind of
      | data except for the magic number and the timestamp that are directly sent to a different RAM in the Output section
  FIFO_data_in : Inport
  FIFO_write_to : Inport  Port=2
  InputState : Inport  Port=3
  data_stream_enable : Inport  Port=4
  RAM address definition : Subsystem
  interpret incoming data : Subsystem
  device_output : Outport
  inc_source_device : Outport  Port=2
  wr_din : Outport  Port=3
  write address : Outport  Port=4
  wr_en : Outport  Port=5
  wires:
  RAM address definition/1(wr_din) -> wr_din/1  "wr_din"
  RAM address definition/2(wr_addr) -> write address/1  "write address"
  FIFO_data_in/1 -> RAM address definition/1(DataIn)
  FIFO_write_to/1 -> interpret incoming data/1(FIFO_write_to), RAM address definition/6(write_to)
  interpret incoming data/5(converter_cnt) -> RAM address definition/5(converter_cnt)
  InputState/1 -> interpret incoming data/2(InputState), RAM address definition/2(InputState)
  interpret incoming data/3(device_output) -> device_output/1
  RAM address definition/3(write_enable_6to15) -> wr_en/1  "wr_en"
  data_stream_enable/1 -> interpret incoming data/3(data_stream_enable)
  interpret incoming data/1(source_device) -> RAM address definition/4(source_device)
  interpret incoming data/2(inc_source_device) -> inc_source_device/1
  interpret incoming data/4(source_channel_0_159) -> RAM address definition/3(source_channel_0_159)

== system gm_CustArch_v2_vnl/cust_architecture_vnl/input_interpret_store_retrieve/store_and_retrieve_input ==
  note: address sent for processing
  note: data sent for processing
  note: reading address
      | from output
  note: current data
  note: current data
  note: Two dual-port RAM for storage and processing
  note: this memory is for synchronizing the current value and
      | the read_from_porcessing_addr since to ouput a value
      | the dual port RAM needs a single clock
  note: writing address
  note: data sent to Output
  read address : Inport
  wr_din : Inport  Port=2
  wr_address : Inport  Port=3
  wr_en : Inport  Port=4
  Memory4 : Memory  InheritSampleTime=on
  Terminator : Terminator
  Terminator6 : Terminator
  input_storage : hdlsllib/HDL RAMs/Dual Port RAM  ram_size=9
      settings: SourceProductBaseCode=SL
  input_storage_for_processing : hdlsllib/HDL RAMs/Dual Port RAM  ram_size=9
      settings: SourceProductBaseCode=SL
  read_from_storage_value : Outport
  current_value : Outport  Port=2
  read_from_porcessing_addr : Outport  Port=3
  wires:
  input_storage_for_processing/2 -> current_value/1  "current value"
  input_storage/2 -> read_from_storage_value/1  "read_from_storage"
  wr_din/1 -> input_storage/1, input_storage_for_processing/1
  input_storage_for_processing/1 -> Terminator6/1
  wr_en/1 -> input_storage/3, input_storage_for_processing/3
  input_storage/1 -> Terminator/1
  read address/1 -> input_storage/4
  wr_address/1 -> input_storage/2, input_storage_for_processing/2, Memory4/1
  Memory4/1 -> input_storage_for_processing/4, read_from_porcessing_addr/1  "read from porcessing addr"

== system gm_CustArch_v2_vnl/cust_architecture_vnl/output_interpret/Interpret_to_RAM_output ==
  OutputState : Inport
  data_stream_en : Inport  Port=2
  Output_State_to_RAM_address (to read) : Subsystem
  "get_enabled_timings " : Subsystem  MinMaxOverflowLogging=MinMaxAndOverflow
  rd_enable : Outport
  read address : Outport  Port=2
  wires:
  Output_State_to_RAM_address (to read)/1(rd_enable) -> rd_enable/1
  data_stream_en/1 -> "get_enabled_timings "/2(data_stream_en)
  OutputState/1 -> "get_enabled_timings "/1(OutputState), Output_State_to_RAM_address (to read)/3(OutputState)
  "get_enabled_timings "/1(source_channel_en) -> Output_State_to_RAM_address (to read)/1(source_channel_en)
  "get_enabled_timings "/2(source_channel_0_159) -> Output_State_to_RAM_address (to read)/2(source_channel_0_159)
  "get_enabled_timings "/3(source_device_enabled) -> Output_State_to_RAM_address (to read)/4(source_device_en)
  Output_State_to_RAM_address (to read)/2(rd_addr) -> read address/1
  "get_enabled_timings "/4(source_device) -> Output_State_to_RAM_address (to read)/5(source_device)
  "get_enabled_timings "/5(converter_cnt) -> Output_State_to_RAM_address (to read)/6(converter_cnt)
